simulink model "Model"  (R2016a)
settings: Solver=VariableStepAuto  StartTime=0.0  StopTime=0  RelTol=1e-3
values from neighbouring files (symbols this model uses):
  disdef = variable(a, 7)    [CollectionAG806_808.m]
  Dpha = 0    [CollectionAG806_808.m]    (also in CourantCCabc.m)
  Dphb = -120    [CollectionAG806_808.m]    (also in CourantCCabc.m)
  Dphc = +120    (= 120)    [CollectionAG806_808.m]    (also in CourantCCabc.m)
  frequence = 60    [CollectionAG806_808.m]    (also in CourantCCabc.m)
  Qc844 = [100e3 100e3 100e3]    [CollectionAG806_808.m]    (also in CourantCCabc.m)
  Qc848 = [150e3 150e3 150e3]    [CollectionAG806_808.m]    (also in CourantCCabc.m)
  RF1 = variable(a, 6)    [CollectionAG806_808.m]
  Ustation = variable(a, 2)    [CollectionAG806_808.m]
  Vstation = variable(a, 1)    [CollectionAG806_808.m]
undefined symbols (not defined in the file or in its folder): activeA, activeB, activeC, C_300, C_301, C_302, C_303, C_304, L_300, L_301, L_302, L_303, L_304, Ltot_806_808, R_300, R_301, R_302, R_303, R_304, reactiveA, reactiveB, reactiveC
libraries: powerlib x311
(part 2 of 2)

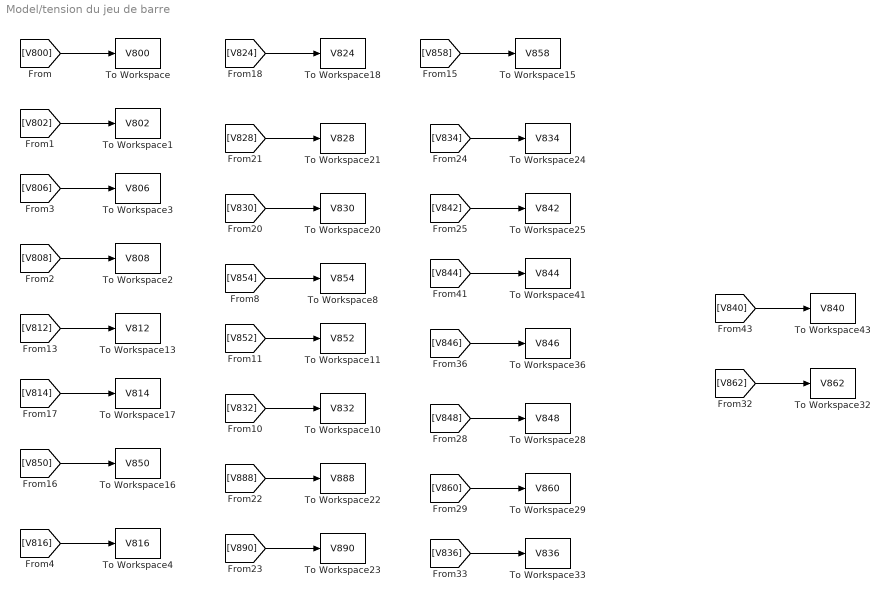
== system Model/tension du jeu de barre ==
  To Workspace : ToWorkspace  VariableName=V800  SampleTime=-1
      settings: Save2DSignal=2-D array (concatenate along first dimension)
  To Workspace1 : ToWorkspace  VariableName=V802  SampleTime=-1
      settings: Save2DSignal=2-D array (concatenate along first dimension)
  To Workspace10 : ToWorkspace  VariableName=V832  SampleTime=-1
      settings: Save2DSignal=2-D array (concatenate along first dimension)
  To Workspace11 : ToWorkspace  VariableName=V852  SampleTime=-1
      settings: Save2DSignal=2-D array (concatenate along first dimension)
  To Workspace13 : ToWorkspace  VariableName=V812  SampleTime=-1
      settings: Save2DSignal=2-D array (concatenate along first dimension)
  To Workspace15 : ToWorkspace  VariableName=V858  SampleTime=-1
      settings: Save2DSignal=2-D array (concatenate along first dimension)
  To Workspace16 : ToWorkspace  VariableName=V850  SampleTime=-1
      settings: Save2DSignal=2-D array (concatenate along first dimension)
  To Workspace17 : ToWorkspace  VariableName=V814  SampleTime=-1
      settings: Save2DSignal=2-D array (concatenate along first dimension)
  To Workspace18 : ToWorkspace  VariableName=V824  SampleTime=-1
      settings: Save2DSignal=2-D array (concatenate along first dimension)
  To Workspace2 : ToWorkspace  VariableName=V808  SampleTime=-1
      settings: Save2DSignal=2-D array (concatenate along first dimension)
  To Workspace20 : ToWorkspace  VariableName=V830  SampleTime=-1
      settings: Save2DSignal=2-D array (concatenate along first dimension)
  To Workspace21 : ToWorkspace  VariableName=V828  SampleTime=-1
      settings: Save2DSignal=2-D array (concatenate along first dimension)
  To Workspace22 : ToWorkspace  VariableName=V888  SampleTime=-1
      settings: Save2DSignal=2-D array (concatenate along first dimension)
  To Workspace23 : ToWorkspace  VariableName=V890  SampleTime=-1
      settings: Save2DSignal=2-D array (concatenate along first dimension)
  To Workspace24 : ToWorkspace  VariableName=V834  SampleTime=-1
      settings: Save2DSignal=2-D array (concatenate along first dimension)
  To Workspace25 : ToWorkspace  VariableName=V842  SampleTime=-1
      settings: Save2DSignal=2-D array (concatenate along first dimension)
  To Workspace28 : ToWorkspace  VariableName=V848  SampleTime=-1
      settings: Save2DSignal=2-D array (concatenate along first dimension)
  To Workspace29 : ToWorkspace  VariableName=V860  SampleTime=-1
      settings: Save2DSignal=2-D array (concatenate along first dimension)
  To Workspace3 : ToWorkspace  VariableName=V806  SampleTime=-1
      settings: Save2DSignal=2-D array (concatenate along first dimension)
  To Workspace32 : ToWorkspace  VariableName=V862  SampleTime=-1
      settings: Save2DSignal=2-D array (concatenate along first dimension)
  To Workspace33 : ToWorkspace  VariableName=V836  SampleTime=-1
      settings: Save2DSignal=2-D array (concatenate along first dimension)
  To Workspace36 : ToWorkspace  VariableName=V846  SampleTime=-1
      settings: Save2DSignal=2-D array (concatenate along first dimension)
  To Workspace4 : ToWorkspace  VariableName=V816  SampleTime=-1
      settings: Save2DSignal=2-D array (concatenate along first dimension)
  To Workspace41 : ToWorkspace  VariableName=V844  SampleTime=-1
      settings: Save2DSignal=2-D array (concatenate along first dimension)
  To Workspace43 : ToWorkspace  VariableName=V840  SampleTime=-1
      settings: Save2DSignal=2-D array (concatenate along first dimension)
  To Workspace8 : ToWorkspace  VariableName=V854  SampleTime=-1
      settings: Save2DSignal=2-D array (concatenate along first dimension)
  wires:
  [V802] -> To Workspace1/1
  [V808] -> To Workspace2/1
  [V806] -> To Workspace3/1
  [V816] -> To Workspace4/1
  [V854] -> To Workspace8/1
  [V832] -> To Workspace10/1
  [V852] -> To Workspace11/1
  [V812] -> To Workspace13/1
  [V850] -> To Workspace16/1
  [V814] -> To Workspace17/1
  [V824] -> To Workspace18/1
  [V830] -> To Workspace20/1
  [V828] -> To Workspace21/1
  [V888] -> To Workspace22/1
  [V890] -> To Workspace23/1
  [V858] -> To Workspace15/1
  [V834] -> To Workspace24/1
  [V842] -> To Workspace25/1
  [V846] -> To Workspace36/1
  [V844] -> To Workspace41/1
  [V840] -> To Workspace43/1
  [V848] -> To Workspace28/1
  [V860] -> To Workspace29/1
  [V862] -> To Workspace32/1
  [V836] -> To Workspace33/1
  [V800] -> To Workspace/1
